simulink model "model_sf_cascade"  (R2016a)
settings: Solver=VariableStepAuto  StartTime=0.0  StopTime=10.0  RelTol=1e-3
values from neighbouring files (symbols this model uses):
  alpha = 0*pi/180    (= 0)    [RunHILsim.m]    (also in RunSimulation.m; plotFrame.m = 0.196349540849; simulation.m)
  b = 0    [Chassis_ss.m]    (also in simulation.m = 0.005)
  c = 0    [Chassis_ss.m]    (also in simulation.m = 0.005)
  g = 9.81    [RunHILsim.m]    (also in RunSimulation.m; simulation.m = 9.82)
  I = 0.007358820323616 - M*l^2    (= 0.00237702032362)    [Chassis_ss.m]    (also in simulation.m = 7.8125e-05)
  J = ML_J + MR_J    (= -8.16854715147e-07)    [Chassis_ss.m]    (also in simulation.m = 3.22e-06)
  l = 95e-3    (= 0.095)    [Chassis_ss.m]    (also in simulation.m = 0.5)
  M = 552e-3    (= 0.552)    [Chassis_ss.m]    (also in simulation.m = 1)
  m = 452e-3    (= 0.452)    [Chassis_ss.m]    (also in simulation.m = 0.5)
  ML_Eta = 0.585848927300825    (= 0.585848927301)    [ControllerDesign.m]
  ML_K = 0.009391068653512    (= 0.00939106865351)    [ControllerDesign.m]
  ML_Kp = 2*ML_L/ML_Tau - ML_R    (= 4.13333333333)    [ControllerDesign.m]
  ML_L = 8.62835e-4    (= 0.000862835)    [ControllerDesign.m]
  ML_N = 30    [ControllerDesign.m]
  ML_R = 6.2    [ControllerDesign.m]
  ML_Tm_neg = -5.830537234675133e-04    (= -0.000583053723468)    [ControllerDesign.m]
  ML_Tm_pos = 6.204835339180699e-04    (= 0.000620483533918)    [ControllerDesign.m]
  MR_Eta = 0.665816712746634    (= 0.665816712747)    [ControllerDesign.m]
  MR_K = 0.009237618864813    (= 0.00923761886481)    [ControllerDesign.m]
  MR_Kp = 2*MR_L/MR_Tau - MR_R    (= 4.46666666667)    [ControllerDesign.m]
  MR_L = 8.62835e-4    (= 0.000862835)    [ControllerDesign.m]
  MR_N = 30    [ControllerDesign.m]
  MR_R = 6.7    [ControllerDesign.m]
  MR_Tm_neg = -5.638334681626818e-04    (= -0.000563833468163)    [ControllerDesign.m]
  MR_Tm_pos = 5.465789021845875e-04    (= 0.000546578902185)    [ControllerDesign.m]
  r = (81.16*10^-3)/2    (= 0.04058)    [Chassis_ss.m]    (also in atan2lookup.m = 1; plotFrame.m = 0.045; simulation.m = 0.045)
  T_motor = 1/200    (= 0.005)    [ControllerDesign.m]
  T_pend = 1/200    (= 0.005)    [ControllerDesign.m]
  theta0 = 25 * pi/180    (= 0.436332312999)    [RunHILsim.m]    (also in RunSimulation.m; simulation.m = 0.0872664625997)
  Vmax = 12    [ControllerDesign.m]
  vref_step_point = 500e-3    (= 0.5)    [RunHILsim.m]    (also in RunSimulation.m)
libraries: cstblocks x3
settings Model: Creator=masom  LastModifiedBy=masom
settings GRTTargetCC: GeneratePreprocessorConditionals=Use local settings

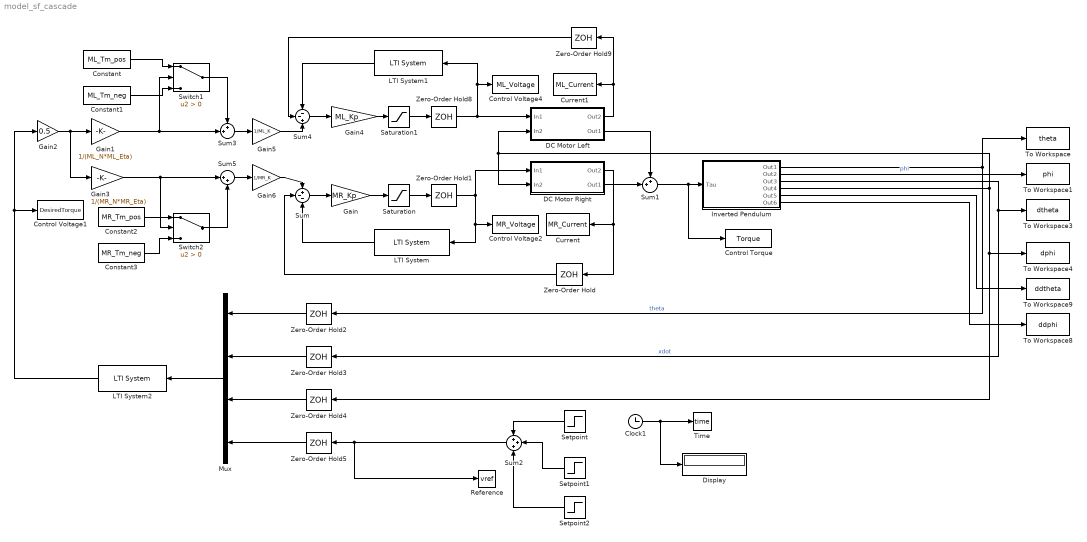
== system model_sf_cascade ==
  Clock1 : Clock
  Constant : Constant  Value=ML_Tm_pos
  Constant1 : Constant  Value=ML_Tm_neg
  Constant2 : Constant  Value=MR_Tm_pos
  Constant3 : Constant  Value=MR_Tm_neg
  Control Torque : ToWorkspace  VariableName=Torque  SaveFormat=Timeseries  SampleTime=-1
  Control Voltage1 : ToWorkspace  VariableName=DesiredTorque  SaveFormat=Timeseries  SampleTime=-1
  Control Voltage2 : ToWorkspace  VariableName=MR_Voltage  SaveFormat=Timeseries  SampleTime=-1
  Control Voltage4 : ToWorkspace  VariableName=ML_Voltage  SaveFormat=Timeseries  SampleTime=-1
  Current : ToWorkspace  VariableName=MR_Current  SampleTime=-1
  Current1 : ToWorkspace  VariableName=ML_Current  SampleTime=-1
  DC Motor Left : Subsystem
  DC Motor Right : Subsystem
  Display : Display
  Gain : Gain  Gain=MR_Kp
  Gain1 : Gain  Gain=1/(ML_N*ML_Eta)
  Gain2 : Gain  Gain=0.5
  Gain3 : Gain  Gain=1/(MR_N*MR_Eta)
  Gain4 : Gain  Gain=ML_Kp
  Gain5 : Gain  Gain=1/ML_K
  Gain6 : Gain  Gain=1/MR_K
  Inverted Pendulum : Subsystem
  LTI System : cstblocks/LTI System  sys=MR_ctrl  IC=[]
  LTI System1 : cstblocks/LTI System  sys=ML_ctrl  IC=[]
  LTI System2 : cstblocks/LTI System  sys=Chassis_ctrl_dss  IC=[]
  Mux : Mux
  Reference : ToWorkspace  VariableName=vref  SampleTime=-1
  Saturation : Saturate  UpperLimit=Vmax  LowerLimit=-Vmax
  Saturation1 : Saturate  UpperLimit=Vmax  LowerLimit=-Vmax
  Setpoint : Step  Time=10  After=vref_step_point  SampleTime=0
  Setpoint1 : Step  Time=11.5  After=-2*vref_step_point  SampleTime=0
  Setpoint2 : Step  Time=20  After=vref_step_point  SampleTime=0
  Sum : Sum  Inputs=+--
  Sum1 : Sum  Inputs=++|
  Sum2 : Sum  Inputs=+++
  Sum3 : Sum  Inputs=++|
  Sum4 : Sum  Inputs=--+
  Sum5 : Sum  Inputs=|++
  Switch1 : Switch  Criteria=u2 > Threshold
  Switch2 : Switch  Criteria=u2 > Threshold
  Time : ToWorkspace  VariableName=time  SampleTime=-1
  To Workspace : ToWorkspace  VariableName=theta  SampleTime=-1
  To Workspace1 : ToWorkspace  VariableName=phi  SampleTime=-1
  To Workspace3 : ToWorkspace  VariableName=dtheta  SampleTime=-1
  To Workspace4 : ToWorkspace  VariableName=dphi  SampleTime=-1
  To Workspace8 : ToWorkspace  VariableName=ddphi  SampleTime=-1
  To Workspace9 : ToWorkspace  VariableName=ddtheta  SampleTime=-1
  Zero-Order Hold{,1,8..9} (4 alike) : ZeroOrderHold  SampleTime=T_motor
  Zero-Order Hold{2..5} (4 alike) : ZeroOrderHold  SampleTime=T_pend
  wires:
  Inverted Pendulum/2(Out2) -> To Workspace1/1  "phi"
  Clock1/1 -> Display/1, Time/1
  Inverted Pendulum/1(Out1) -> Zero-Order Hold2/1, To Workspace/1  "theta"
  Setpoint/1 -> Sum2/1
  Setpoint1/1 -> Sum2/2
  Sum2/1 -> Reference/1, Zero-Order Hold5/1
  Inverted Pendulum/3(Out3) -> To Workspace3/1, Zero-Order Hold3/1  "xdot"
  Inverted Pendulum/5(Out5) -> To Workspace9/1
  Inverted Pendulum/6(Out6) -> To Workspace8/1
  Inverted Pendulum/4(Out4) -> To Workspace4/1, Zero-Order Hold4/1, DC Motor Left/2(In2), DC Motor Right/2(In2)
  DC Motor Right/2(Out1) -> Sum1/2
  DC Motor Right/1(Out2) -> Zero-Order Hold/1, Current/1
  Zero-Order Hold/1 -> Sum/2
  Sum/1 -> Gain/1
  Saturation/1 -> Zero-Order Hold1/1
  LTI System/1 -> Sum/3
  Zero-Order Hold1/1 -> LTI System/1, Control Voltage2/1, DC Motor Right/1(In1)
  Gain3/1 -> Sum5/1, Switch2/2
  Setpoint2/1 -> Sum2/3
  DC Motor Left/2(Out1) -> Sum1/1
  Zero-Order Hold8/1 -> DC Motor Left/1(In1), LTI System1/1, Control Voltage4/1
  Saturation1/1 -> Zero-Order Hold8/1
  Gain4/1 -> Saturation1/1
  Sum3/1 -> Gain5/1
  Sum4/1 -> Gain4/1
  LTI System1/1 -> Sum4/1
  DC Motor Left/1(Out2) -> Zero-Order Hold9/1, Current1/1
  Zero-Order Hold9/1 -> Sum4/2
  Mux/1 -> LTI System2/1
  Zero-Order Hold2/1 -> Mux/1
  Zero-Order Hold3/1 -> Mux/2
  Zero-Order Hold4/1 -> Mux/3
  Zero-Order Hold5/1 -> Mux/4
  LTI System2/1 -> Control Voltage1/1, Gain2/1
  Gain2/1 -> Gain1/1, Gain3/1
  Gain/1 -> Saturation/1
  Sum1/1 -> Control Torque/1, Inverted Pendulum/1(Tau)
  Gain1/1 -> Sum3/2, Switch1/2
  Constant/1 -> Switch1/1
  Constant1/1 -> Switch1/3
  Constant2/1 -> Switch2/1
  Constant3/1 -> Switch2/3
  Sum5/1 -> Gain6/1
  Gain5/1 -> Sum4/3
  Gain6/1 -> Sum/1
  Switch1/1 -> Sum3/1
  Switch2/1 -> Sum5/2

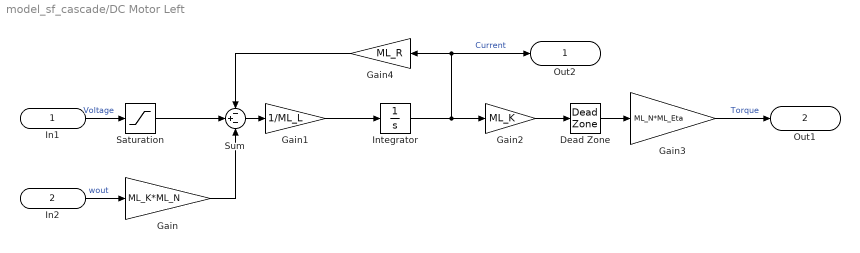
== system model_sf_cascade/DC Motor Left ==
  In1 : Inport
  In2 : Inport  Port=2
  Dead Zone : DeadZone  LowerValue=MR_Tm_neg  UpperValue=MR_Tm_pos  SaturateOnIntegerOverflow=on
  Gain : Gain  Gain=ML_K*ML_N
  Gain1 : Gain  Gain=1/ML_L
  Gain2 : Gain  Gain=ML_K
  Gain3 : Gain  Gain=ML_N*ML_Eta
  Gain4 : Gain  Gain=ML_R
  Integrator : Integrator
  Saturation : Saturate  UpperLimit=Vmax  LowerLimit=-Vmax
  Sum : Sum  Inputs=-+-
  Out2 : Outport
  Out1 : Outport  Port=2
  wires:
  Saturation/1 -> Sum/2
  Gain4/1 -> Sum/1
  Integrator/1 -> Gain2/1, Out2/1, Gain4/1  "Current"
  Gain3/1 -> Out1/1  "Torque"
  Dead Zone/1 -> Gain3/1
  Gain2/1 -> Dead Zone/1
  Gain1/1 -> Integrator/1
  Sum/1 -> Gain1/1
  Gain/1 -> Sum/3
  In2/1 -> Gain/1  "wout"
  In1/1 -> Saturation/1  "Voltage"

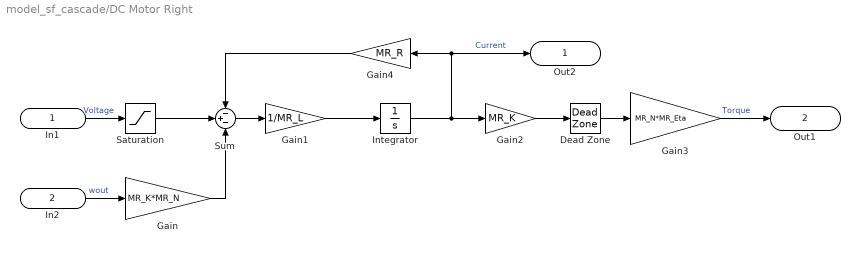
== system model_sf_cascade/DC Motor Right ==
  In1 : Inport
  In2 : Inport  Port=2
  Dead Zone : DeadZone  LowerValue=MR_Tm_neg  UpperValue=MR_Tm_pos  SaturateOnIntegerOverflow=on
  Gain : Gain  Gain=MR_K*MR_N
  Gain1 : Gain  Gain=1/MR_L
  Gain2 : Gain  Gain=MR_K
  Gain3 : Gain  Gain=MR_N*MR_Eta
  Gain4 : Gain  Gain=MR_R
  Integrator : Integrator
  Saturation : Saturate  UpperLimit=Vmax  LowerLimit=-Vmax
  Sum : Sum  Inputs=-+-
  Out2 : Outport
  Out1 : Outport  Port=2
  wires:
  In1/1 -> Saturation/1  "Voltage"
  In2/1 -> Gain/1  "wout"
  Gain/1 -> Sum/3
  Sum/1 -> Gain1/1
  Gain1/1 -> Integrator/1
  Gain2/1 -> Dead Zone/1
  Dead Zone/1 -> Gain3/1
  Gain3/1 -> Out1/1  "Torque"
  Integrator/1 -> Gain4/1, Out2/1, Gain2/1  "Current"
  Gain4/1 -> Sum/1
  Saturation/1 -> Sum/2

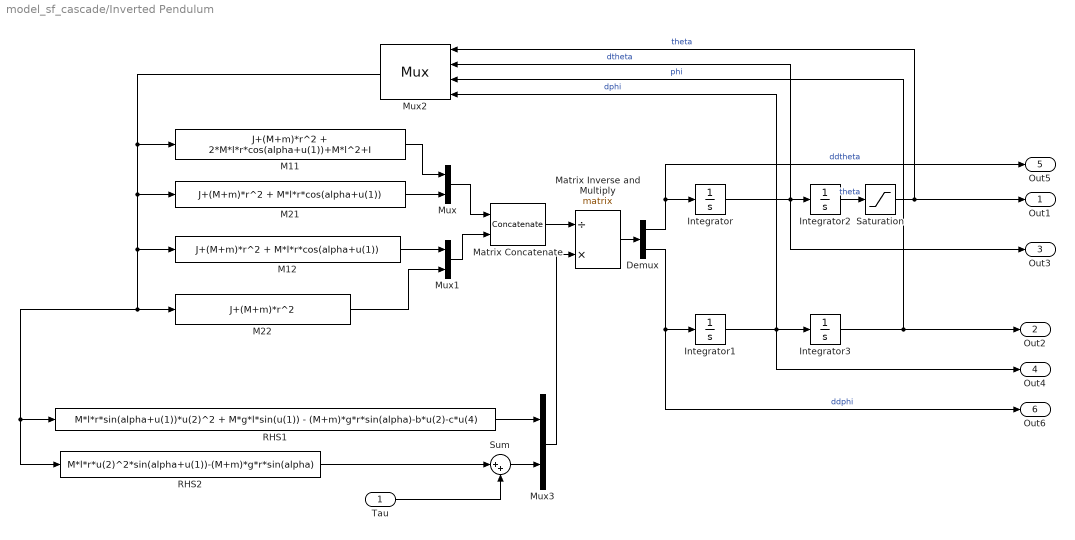
== system model_sf_cascade/Inverted Pendulum ==
  Tau : Inport
  Demux : Demux  Outputs=2
  Integrator : Integrator  ContinuousStateAttributes='dtheta'
  Integrator1 : Integrator  ContinuousStateAttributes='dphi'
  Integrator2 : Integrator  InitialCondition=theta0  ContinuousStateAttributes='theta'
  Integrator3 : Integrator  ContinuousStateAttributes='phi'
  M11 : Fcn  Expr=J+(M+m)*r^2 + 2*M*l*r*cos(alpha+u(1))+M*l^2+I
  M12 : Fcn  Expr=J+(M+m)*r^2 + M*l*r*cos(alpha+u(1))
  "M21 " : Fcn  Expr=J+(M+m)*r^2 + M*l*r*cos(alpha+u(1))
  M22 : Fcn  Expr=J+(M+m)*r^2
  Matrix Concatenate : Concatenate  Mode=Multidimensional array  ConcatenateDimension=2
  Matrix Inverse and Multiply : Product  Inputs=/*  Multiplication=Matrix(*)
  Mux : Mux  Inputs=2
  Mux1 : Mux  Inputs=2
  Mux2 : Mux
      settings: DisplayOption=signals
  Mux3 : Mux  Inputs=2
  RHS1 : Fcn  Expr=M*l*r*sin(alpha+u(1))*u(2)^2 + M*g*l*sin(u(1)) - (M+m)*g*r*sin(alpha)-b*u(2)-c*u(4)
  RHS2 : Fcn  Expr=M*l*r*u(2)^2*sin(alpha+u(1))-(M+m)*g*r*sin(alpha)
  Saturation : Saturate  UpperLimit=pi  LowerLimit=-pi
  Sum : Sum  Inputs=|++
  Out1 : Outport
  Out2 : Outport  Port=2
  Out3 : Outport  Port=3
  Out4 : Outport  Port=4
  Out5 : Outport  Port=5
  Out6 : Outport  Port=6
  wires:
  M12/1 -> Mux1/1
  Integrator1/1 -> Out4/1, Mux2/4, Integrator3/1  "dphi"
  Demux/1 -> Out5/1, Integrator/1  "ddtheta"
  Mux/1 -> Matrix Concatenate/1
  Matrix Concatenate/1 -> Matrix Inverse and Multiply/1
  Demux/2 -> Integrator1/1, Out6/1  "ddphi"
  Mux1/1 -> Matrix Concatenate/2
  RHS2/1 -> Sum/1
  Matrix Inverse and Multiply/1 -> Demux/1
  Sum/1 -> Mux3/2
  Integrator/1 -> Out3/1, Mux2/2, Integrator2/1  "dtheta"
  Integrator2/1 -> Saturation/1  "theta"
  Mux2/1 -> "M21 "/1, M22/1, RHS2/1, RHS1/1, M12/1, M11/1
  Mux3/1 -> Matrix Inverse and Multiply/2
  M11/1 -> Mux/1
  "M21 "/1 -> Mux/2
  Integrator3/1 -> Out2/1, Mux2/3  "phi"
  RHS1/1 -> Mux3/1
  Tau/1 -> Sum/2
  M22/1 -> Mux1/2
  Saturation/1 -> Out1/1, Mux2/1  "theta"
